simulink model "Application_BMS"  (R2024b)
settings: Solver=FixedStepDiscrete  StartTime=0.0  StopTime=660  FixedStep=BMSk_stepSize  RelTol=1e-3  EnableMultiTasking=on
values from neighbouring files (symbols this model uses):
  BMSc_airTemperature = air_temperature    (= 35)    [BMS_init.m]
  BMSc_cabinTemperature = 25    [BMS_init.m]
  BMSk_stepSize = 0.1    [BMS_init.m]
settings Model: PauseTimes=22  Creator=ms2zwt  LastModifiedBy=voillat
settings ConfigSet: Description=OpenECU configuration set for code generation under RTW-EC.
settings SolverCC: AlgebraicLoopSolver=TrustRegion  PositivePriorityOrder=on
settings DataIOCC: LimitDataPoints=on  SaveFormat=Array  SignalLoggingSaveFormat=ModelDataLogs
settings OptimizationCC: DefaultParameterBehavior=Inlined  InlineInvariantSignals=on  ExpressionDepthLimit=2147483647  StateBitsets=on  DataBitsets=on  ZeroExternalMemoryAtStartup=off  ZeroInternalMemoryAtStartup=off  NoFixptDivByZeroProtection=on  EfficientFloat2IntCast=on  LifeSpan=1  EfficientTunableParamExpr=on
settings DebuggingCC: SaveWithParameterizedLinksMsg=none  SignalResolutionControl=TryResolveAllWithWarning  MultiTaskDSMMsg=warning  MultiTaskCondExecSysMsg=none  SingleTaskRateTransMsg=error  CheckMatrixSingularityMsg=warning  VectorMatrixConversionMsg=warning  SignalLabelMismatchMsg=warning  UnconnectedInputMsg=warning  UnconnectedOutputMsg=warning  UnconnectedLineMsg=warning  AllowSymbolicDim=off  StateNameClashWarn=warning  SFUnexpectedBacktrackingDiag=warning  SFNoUnconditionalDefaultTransitionDiag=warning  SFExecutionAtInitializationDiag=none  ArithmeticOperatorsInVariantConditions=warning
settings HardwareCC: ProdBitPerPointer=32  ProdBitPerSizeT=32  ProdBitPerPtrDiffT=32  ProdLargestAtomicInteger=Long  ProdLargestAtomicFloat=Double  ProdEndianess=BigEndian  ProdWordSize=32  ProdHWDeviceType=Freescale->32-bit PowerPC  TargetIntDivRoundTo=Zero  TargetEndianess=BigEndian  TargetHWDeviceType=Freescale->32-bit PowerPC  ProdEqTarget=off
settings ModelReferenceCC: EnableRefExpFcnMdlSchedulingChecks=on  PropagateSignalLabelsOutOfModel=off
settings SFSimCC: SimUseLocalCustomCode=off  MATLABDynamicMemAlloc=off  CustomCodeUndefinedFunction=UseInterfaceOnly
settings RTWCC: Description=OpenECU Platform Target (ERT, optimised floating-point code)  SystemTargetFile=openecu_ert.tlc  MakeCommand=make_rtw optimized_floating_point=1  TemplateMakefile=openecu_ert_r2015b_64.tmf  RetainRTWFile=on  RTWUseLocalCustomCode=off  IncludeHyperlinkInReport=on  GPUComputeCapability=3.5
settings CodeAppCC: ForceParamTrailComments=on  IgnoreCustomStorageClasses=off  SimulinkDataObjDesc=on  CustomSymbolStrType=$N$R$M  InsertBlockDesc=on  StateflowObjectComments=on  InternalIdentifier=Classic
settings STFCustomTargetCC: TargetLibSuffix=.a  GenerateSampleERTMain=on  IncludeMdlTerminateFcn=off  CombineOutputUpdateFcns=on  IncludeFileDelimiter=UseQuote  ERTCustomFileBanners=on  SupportContinuousTime=off  RemoveResetFunc=on  MATLABClassNameForMDSCustomization=Simulink.SoftwareTarget.ERTCustomization  SystemTargetFile=openecu_ert.tlc
settings ERTTargetCC: MultiwordLength=2048  GenerateSampleERTMain=on  ParMdlRefBuildCompliant=off  CompOptLevelCompliant=off  ConcurrentExecutionCompliant=off  IncludeMdlTerminateFcn=off  IncludeFileDelimiter=UseQuote  SupportNonInlinedSFcns=on  ModelStepFunctionPrototypeControlCompliant=off  CPPClassGenCompliant=off  UseToolchainInfoCompliant=off  ExtModeMexFile=noextcomm  ERTSrcFileBannerTemplate=oe_code_c_template.cgt  ERTHdrFileBannerTemplate=oe_code_h_template.cgt  ERTDataSrcFileTemplate=oe_data_c_template.cgt  ERTDataHdrFileTemplate=oe_data_h_template.cgt  ERTCustomFileTemplate=example_file_process.tlc  GlobalDataDefinition=InSeparateSourceFile  GlobalDataReference=InSeparateHeaderFile  ConvertIfToSwitch=off  SuppressUnreachableDefaultCases=off  EnableUserReplacementTypes=on  DynamicArrayContainerType=coder::array
settings ConfigComp: CovMetricSettings=dw  CovSaveCumulativeToWorkspaceVar=on  CovSaveSingleToWorkspaceVar=on  CovExternalEMLEnable=off

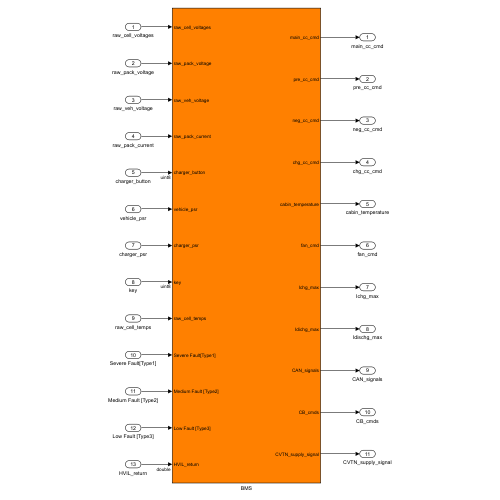
[thumbnail: Simulink's stored preview of the top-level diagram]
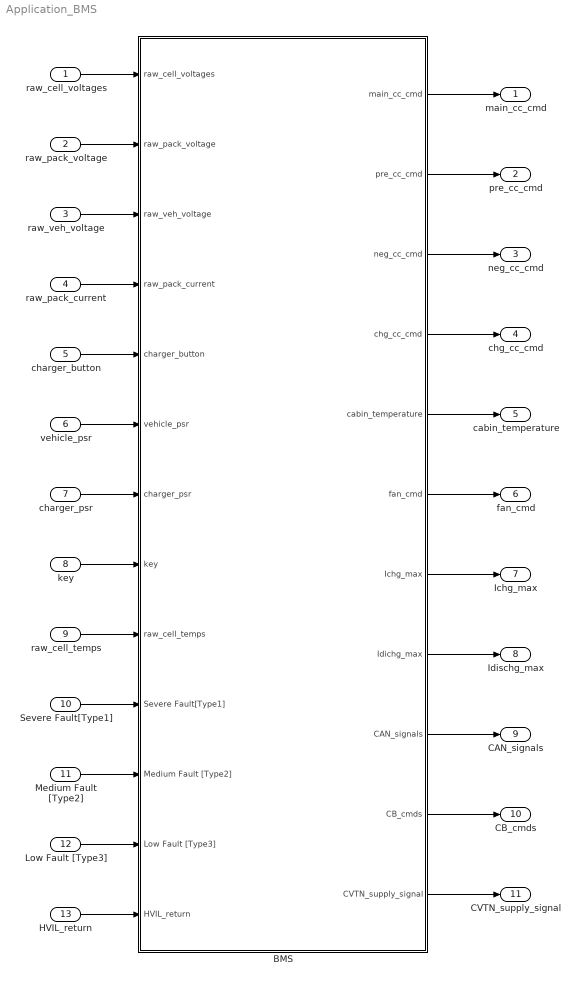
== system Application_BMS ==
  raw_cell_voltages : Inport
  raw_pack_voltage : Inport  Port=2
  raw_veh_voltage : Inport  Port=3
  raw_pack_current : Inport  Port=4
  charger_button : Inport  Port=5
  vehicle_psr : Inport  Port=6
  charger_psr : Inport  Port=7
  key : Inport  Port=8
  raw_cell_temps : Inport  Port=9
  Severe Fault[Type1] : Inport  Port=10
  Medium Fault [Type2] : Inport  Port=11
  Low Fault [Type3] : Inport  Port=12
  HVIL_return : Inport  Port=13
  BMS : Subsystem
  main_cc_cmd : Outport  VectorParamsAs1DForOutWhenUnconnected=off
  pre_cc_cmd : Outport  Port=2  VectorParamsAs1DForOutWhenUnconnected=off
  neg_cc_cmd : Outport  Port=3  VectorParamsAs1DForOutWhenUnconnected=off
  chg_cc_cmd : Outport  Port=4  VectorParamsAs1DForOutWhenUnconnected=off
  cabin_temperature : Outport  Port=5  VectorParamsAs1DForOutWhenUnconnected=off
  fan_cmd : Outport  Port=6  VectorParamsAs1DForOutWhenUnconnected=off
  Ichg_max : Outport  Port=7  VectorParamsAs1DForOutWhenUnconnected=off
  Idischg_max : Outport  Port=8  VectorParamsAs1DForOutWhenUnconnected=off
  CAN_signals : Outport  Port=9  VectorParamsAs1DForOutWhenUnconnected=off
  CB_cmds : Outport  Port=10  VectorParamsAs1DForOutWhenUnconnected=off
  CVTN_supply_signal : Outport  Port=11  VectorParamsAs1DForOutWhenUnconnected=off
  wires:
  raw_cell_voltages/1 -> BMS/1(raw_cell_voltages)
  raw_pack_voltage/1 -> BMS/2(raw_pack_voltage)
  raw_veh_voltage/1 -> BMS/3(raw_veh_voltage)
  raw_pack_current/1 -> BMS/4(raw_pack_current)
  charger_button/1 -> BMS/5(charger_button)
  vehicle_psr/1 -> BMS/6(vehicle_psr)
  charger_psr/1 -> BMS/7(charger_psr)
  key/1 -> BMS/8(key)
  raw_cell_temps/1 -> BMS/9(raw_cell_temps)
  Severe Fault[Type1]/1 -> BMS/10(Severe Fault[Type1])
  Medium Fault [Type2]/1 -> BMS/11(Medium Fault [Type2])
  Low Fault [Type3]/1 -> BMS/12(Low Fault [Type3])
  HVIL_return/1 -> BMS/13(HVIL_return)
  BMS/1(main_cc_cmd) -> main_cc_cmd/1
  BMS/2(pre_cc_cmd) -> pre_cc_cmd/1
  BMS/3(neg_cc_cmd) -> neg_cc_cmd/1
  BMS/4(chg_cc_cmd) -> chg_cc_cmd/1
  BMS/5(cabin_temperature) -> cabin_temperature/1
  BMS/6(fan_cmd) -> fan_cmd/1
  BMS/7(Ichg_max) -> Ichg_max/1
  BMS/8(Idichg_max) -> Idischg_max/1
  BMS/9(CAN_signals) -> CAN_signals/1
  BMS/10(CB_cmds) -> CB_cmds/1
  BMS/11(CVTN_supply_signal) -> CVTN_supply_signal/1

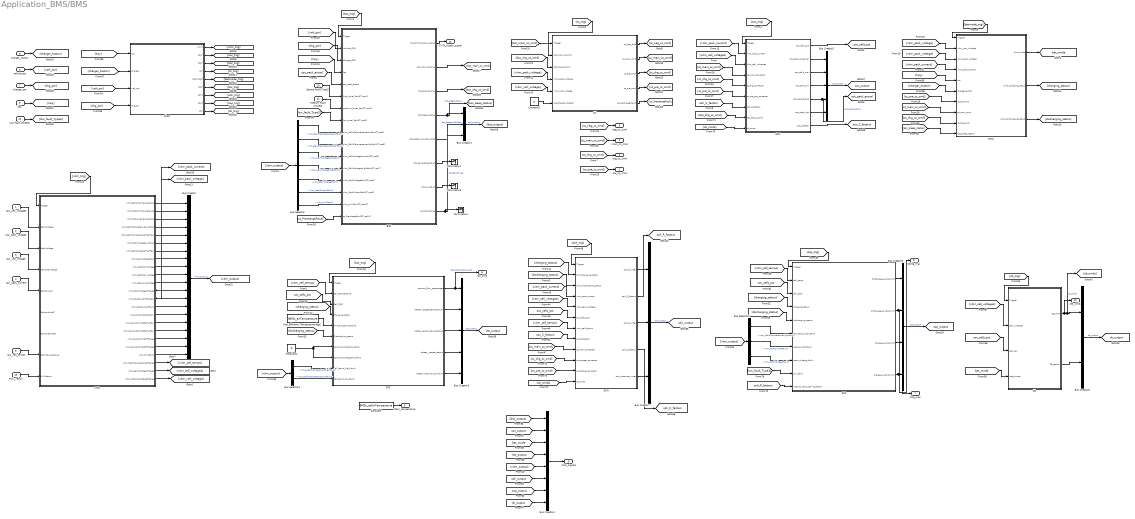
== system Application_BMS/BMS ==
  raw_cell_voltages : Inport
  raw_pack_voltage : Inport  Port=2
  raw_veh_voltage : Inport  Port=3
  raw_pack_current : Inport  Port=4
  charger_button : Inport  Port=5  OutDataTypeStr=uint8
  vehicle_psr : Inport  Port=6
  charger_psr : Inport  Port=7
  key : Inport  Port=8  OutDataTypeStr=uint8
  raw_cell_temps : Inport  Port=9
  Severe Fault[Type1] : Inport  Port=10
  Medium Fault [Type2] : Inport  Port=11
  Low Fault [Type3] : Inport  Port=12
  HVIL_return : Inport  Port=13  OutDataTypeStr=double
  BMO : Subsystem  Variant=on
  BSC : Subsystem  Variant=on
  BTC : Subsystem  Variant=on
  Bus Creator : BusCreator  Inputs=20
  Bus Creator1 : BusCreator  Inputs=3
  Bus Creator2 : BusCreator  Inputs=5
  Bus Creator3 : BusCreator  Inputs=5
  Bus Creator4 : BusCreator  Inputs=8
  Bus Creator5 : BusCreator  Inputs=4
  Bus Creator6 : BusCreator  Inputs=2
  Bus Creator7 : BusCreator  Inputs=3
  Bus Selector : BusSelector  OutputSignals=vitm_CellsTemperatureLowFault,vitm_CellsTemperatureHighFault,vitm_CellsVoltageLowFault,vitm_CellsVoltageHighFault,vitm_PackVoltageFault,vitm_PackCurrentFault,vitm_HVILFault
  Bus Selector1 : BusSelector  OutputSignals=vitm_CellsTemperatureHighFault,vitm_CellsTemperatureLowFault
  Bus Selector2 : BusSelector  OutputSignals=vitm_CellsTemperatureHighFault,vitm_PackCurrentFault,vitm_PackVoltageFault
  CB : Subsystem  Variant=on
  CC : Subsystem  Variant=on
  Chart : Stateflow chart  TreatAsAtomicUnit=on
  Constant : Constant  Value=BMSc_cabinTemperature  SampleTime=BMSk_stepSize
  Constant1 : Constant  Value=0  OutDataTypeStr=boolean  SampleTime=-1
  Constant2 : Constant  Value=0  OutDataTypeStr=double  SampleTime=-1
  Max Efficiency Temperature degC : Constant  Value=BMSc_airTemperature  SampleTime=BMSk_stepSize
  SOC : Subsystem  Variant=on
  SOH : Subsystem  Variant=on
  SOP : Subsystem  Variant=on
  Terminator1 : Terminator
  Terminator3 : Terminator
  Terminator4 : Terminator
  VITM : Subsystem  Variant=on
  main_cc_cmd : Outport  VectorParamsAs1DForOutWhenUnconnected=off
  pre_cc_cmd : Outport  Port=2  VectorParamsAs1DForOutWhenUnconnected=off
  neg_cc_cmd : Outport  Port=3  VectorParamsAs1DForOutWhenUnconnected=off
  chg_cc_cmd : Outport  Port=4  VectorParamsAs1DForOutWhenUnconnected=off
  cabin_temperature : Outport  Port=5  VectorParamsAs1DForOutWhenUnconnected=off
  fan_cmd : Outport  Port=6  VectorParamsAs1DForOutWhenUnconnected=off
  Ichg_max : Outport  Port=7  VectorParamsAs1DForOutWhenUnconnected=off
  Idichg_max : Outport  Port=8  VectorParamsAs1DForOutWhenUnconnected=off
  CAN_signals : Outport  Port=9  VectorParamsAs1DForOutWhenUnconnected=off
  CB_cmds : Outport  Port=10  VectorParamsAs1DForOutWhenUnconnected=off
  CVTN_supply_signal : Outport  Port=11  VectorParamsAs1DForOutWhenUnconnected=off
  tag scope: bat_mode=global, btc_output=global, cb_output=global, soc_C_factors=global, soc_cells_pct=global, soc_output=global, soc_pack_actual=global, soh_C_factors=global, soh_R_factors=global, soh_output=global, sop_output=global
  wires:
  Chart/1(vitm()) -> [vitm_trig]
  Chart/2(soc()) -> [soc_trig]
  Chart/3(bsc()) -> [bsc_trig]
  Chart/4(cc()) -> [cc_trig]
  Chart/5(batmode()) -> [batmode_trig]
  Constant/1 -> cabin_temperature/1
  [cc_neg_cc_cmd] -> neg_cc_cmd/1
  [cc_main_cc_cmd] -> main_cc_cmd/1
  [cc_chg_cc_cmd] -> chg_cc_cmd/1
  [cc_pre_cc_cmd] -> pre_cc_cmd/1
  Chart/6(btc()) -> [btc_trig]
  Bus Creator/1 -> [vitm_output]  "vitm_output"
  [vitm_output] -> Bus Selector/1
  charger_button/1 -> [charger_button]
  vehicle_psr/1 -> [veh_psr]
  [veh_psr] -> Chart/3(veh_psr)
  [vitm_output] -> Bus Selector1/1
  Bus Creator1/1 -> [bsc_output]  "bsc_output"
  Bus Creator2/1 -> [soc_output]  "soc_output"
  Bus Creator3/1 -> [btc_output]  "btc_output"
  [bsc_output] -> Bus Creator4/1
  [soc_output] -> Bus Creator4/2
  [bat_mode] -> Bus Creator4/3
  [btc_output] -> Bus Creator4/4
  [vitm_output] -> Bus Creator4/5
  Bus Creator4/1 -> CAN_signals/1
  Chart/7(soh()) -> [soh_trig]
  Chart/8(sop()) -> [sop_trig]
  [vitm_output] -> Bus Selector2/1
  Chart/9(cb()) -> [cb_trig]
  Bus Creator5/1 -> [sop_output]  "sop_output"
  [sop_output] -> Bus Creator4/7
  charger_psr/1 -> [chg_psr]
  [chg_psr] -> Chart/4(chg_psr)
  key/1 -> [key]
  [charger_button] -> Chart/2(charger)
  [key] -> Chart/1(key)
  Bus Creator6/1 -> [cb_output]  "cb_output"
  [cb_output] -> Bus Creator4/8
  Bus Creator7/1 -> [soh_output]  "soh_output"
  [soh_output] -> Bus Creator4/6
  Low Fault [Type3]/1 -> [low_fault_Type3]
  [vitm_pack_voltage] -> BMO/2(vitm_veh_voltage)
  [vitm_pack_voltage] -> BMO/3(vitm_pack_voltage)
  [vitm_pack_current] -> BMO/4(vitm_pack_current)
  [key] -> BMO/5(key)
  [charger_button] -> BMO/6(charger_button)
  [cc_pre_cc_cmd] -> BMO/7(cc_pre_cmd)
  [cc_main_cc_cmd] -> BMO/8(cc_main_cmd)
  [cc_chg_cc_cmd] -> BMO/9(cc_chg_cmd)
  [bsc_sleep_status] -> BMO/10(bsc_sleep_status)
  [batmode_trig] -> BMO/1(Trigger)
  BMO/1(bmo_mode) -> [bat_mode]
  BMO/2(bmo_charging_status) -> [charging_status]
  BMO/3(bmo_discharging_status) -> [discharging_status]
  [veh_psr] -> BSC/2(vehicle_PSR)
  [chg_psr] -> BSC/3(charger_PSR)
  [key] -> BSC/4(key)
  [soc_pack_actual] -> BSC/5(soc_pack_actual)
  Severe Fault[Type1]/1 -> BSC/6(high_level_fault[Type1])
  Medium Fault [Type2]/1 -> BSC/7(medium_level_fault[Type2])
  [low_fault_Type3] -> BSC/8(low_level_fault[Type3])
  Bus Selector/1 -> BSC/9(vitm_CellsTemperatureLowFault[Type4])  "<vitm_CellsTemperatureLowFault>"
  Bus Selector/2 -> BSC/10(vitm_CellsTemperatureHighFault[Type5])  "<vitm_CellsTemperatureHighFault>"
  Bus Selector/3 -> BSC/11(vitm_CellsVoltageLowFault[Type6])  "<vitm_CellsVoltageLowFault>"
  Bus Selector/4 -> BSC/12(vitm_CellsVoltageHightFault[Type7])  "<vitm_CellsVoltageHighFault>"
  Bus Selector/5 -> BSC/13(vitm_PackVoltageFault[Type8])  "<vitm_PackVoltageFault>"
  Bus Selector/6 -> BSC/14(vitm_PackCurrentFault[Type9])  "<vitm_PackCurrentFault>"
  Bus Selector/7 -> BSC/15(vitm_HVILFault[Type10])  "<vitm_HVILFault>"
  [cc_PrechargeFault] -> BSC/16(cc_PrechargeFault[Type11])
  [bsc_trig] -> BSC/1(Trigger)
  BSC/1(bsc_CVTN_supply_signal) -> CVTN_supply_signal/1
  BSC/2(bsc_main_cc_cmd) -> [bsc_main_cc_cmd]
  BSC/3(bsc_chg_cc_cmd) -> [bsc_chg_cc_cmd]
  BSC/4(bsc_sleep_status) -> Bus Creator1/1, [bsc_sleep_status]  "bsc_sleep_status"
  BSC/5(bsc_reason_to_open_CAN) -> Bus Creator1/2  "bsc_ReasonToOpen"
  BSC/6(bsc_severemed_fault) -> Terminator1/1
  BSC/7(bsc_low_fault) -> Terminator3/1
  BSC/8(bsc_fault_type) -> Terminator4/1, Bus Creator1/3  "bsc_FaultType"
  [vitm_cell_temps] -> BTC/2(Cell_temperature)
  [soc_cells_pct] -> BTC/3(Cell_SOC)
  [charging_status] -> BTC/4(Charging_status)
  Max Efficiency Temperature degC/1 -> BTC/5(Ambient_temperature)
  [discharging_status] -> BTC/6(Discharging_status)
  Constant1/1 -> BTC/7(Coolant_inlet_temp_fault), BTC/8(Coolant_outlet_temp_fault)
  Bus Selector1/1 -> BTC/9(Cell_temp_high_fault)  "<vitm_CellsTemperatureHighFault>"
  Bus Selector1/2 -> BTC/10(Cell_temp_low_fault)  "<vitm_CellsTemperatureLowFault>"
  [btc_trig] -> BTC/1(Trigger)
  BTC/1(coolant_flow_percentage) -> Bus Creator3/1, fan_cmd/1  "btc_coolant_flow_pct"
  BTC/2(battery_target_temperature) -> Bus Creator3/2
  BTC/3(battery_actual_temperature) -> Bus Creator3/3
  BTC/4(battery_reqest_status) -> Bus Creator3/4
  BTC/5(battery_thermal_condition) -> Bus Creator3/5
  [vitm_cell_voltages] -> CB/2(cell_voltages)
  [soc_cells_pct] -> CB/3(cell_soc)
  [bat_mode] -> CB/4(batt_mode)
  [cb_trig] -> CB/1(Trigger)
  CB/1(CB_cmd) -> [cb_cmds], Bus Creator6/1, CB_cmds/1  "cb_cmds"
  CB/2(CB_status) -> Bus Creator6/2
  [bsc_main_cc_cmd] -> CC/2(bsc_main_cc_cmd)
  [bsc_chg_cc_cmd] -> CC/3(bsc_chg_cc_cmd)
  [vitm_pack_voltage] -> CC/4(vitm_pack_voltage)
  [vitm_veh_voltage] -> CC/5(vitm_veh_voltage)
  Constant2/1 -> CC/6(pre_chg_fault_reset)
  [cc_trig] -> CC/1(Trigger)
  CC/1(cc_neg_cmd) -> [cc_neg_cc_cmd]
  CC/2(cc_main_cmd) -> [cc_main_cc_cmd]
  CC/3(cc_chg_cmd) -> [cc_chg_cc_cmd]
  CC/4(cc_pre_cmd) -> [cc_pre_cc_cmd]
  CC/5(cc_precharge_fault) -> [cc_PrechargeFault]
  [vitm_pack_current] -> SOC/2(vitm_pack_current)
  [vitm_cell_voltages] -> SOC/3(vitm_cell_voltages)
  [cc_main_cc_cmd] -> SOC/4(cc_main_contactor)
  [cc_chg_cc_cmd] -> SOC/5(cc_chg_contactor)
  [cc_pre_cc_cmd] -> SOC/6(cc_pre_chg_contactor)
  [soh_C_factors] -> SOC/7(soh_C_factors)
  [bsc_chg_cc_cmd] -> SOC/8(bsc_chg_cc_cmd)
  [cb_cmds] -> SOC/9(cb_cmds)
  [soc_trig] -> SOC/1(Trigger)
  SOC/1(soc_cells_pct) -> [soc_cells_pct]
  SOC/2(soc_pack_customer) -> Bus Creator2/1
  SOC/3(soc_cells_max) -> Bus Creator2/2
  SOC/4(soc_cells_min) -> Bus Creator2/3
  SOC/5(soc_pack_actual) -> [soc_pack_actual], Bus Creator2/4  "soc_pack_actual"
  SOC/6(soc_rate_high) -> Bus Creator2/5
  SOC/7(soc_C_factor) -> [soc_C_factors]
  [charging_status] -> SOH/2(bmo_charging_status)
  [discharging_status] -> SOH/3(bmo_discharging_status)
  [vitm_pack_current] -> SOH/4(vitm_pack_current)
  [vitm_cell_voltages] -> SOH/5(vitm_cell_voltages)
  [soc_cells_pct] -> SOH/6(soc_cells_pct)
  [vitm_cell_temps] -> SOH/7(vitm_cells_temp)
  [soc_C_factors] -> SOH/8(soc_C_factors)
  [cc_main_cc_cmd] -> SOH/9(cc_main_contactor)
  [cc_chg_cc_cmd] -> SOH/10(cc_charger_contactor)
  [cc_pre_cc_cmd] -> SOH/11(cc_prechg_contactor)
  [cb_cmds] -> SOH/12(cb_cmds)
  [soh_trig] -> SOH/1(Trigger)
  SOH/1(soh_R_index) -> Bus Creator7/1
  SOH/2(soh_R_factors) -> [soh_R_factors]
  SOH/3(soh_C_index) -> Bus Creator7/2
  SOH/4(soh_C_factors) -> [soh_C_factors]
  SOH/5(soh_customer_index) -> Bus Creator7/3
  [vitm_cell_temps] -> SOP/2(cell_temp)
  [soc_cells_pct] -> SOP/3(cell_SOC)
  [charging_status] -> SOP/4(charging_status)
  [discharging_status] -> SOP/5(discharging_status)
  Bus Selector2/1 -> SOP/6(cell_temp_high_Fault)  "<vitm_CellsTemperatureHighFault>"
  Bus Selector2/2 -> SOP/7(pack_current_fault)  "<vitm_PackCurrentFault>"
  Bus Selector2/3 -> SOP/8(pack_voltage_fault)  "<vitm_PackVoltageFault>"
  [low_fault_Type3] -> SOP/9(low_fault)
  [soh_R_factors] -> SOP/10(internal_resis_scaling_factor)
  [sop_trig] -> SOP/1(Trigger)
  SOP/1(discharge_power_limit) -> Bus Creator5/1
  SOP/2(discharge_current_limit) -> Idichg_max/1, Bus Creator5/2
  SOP/3(charge_power_limit) -> Bus Creator5/3
  SOP/4(charge_current_limit) -> Bus Creator5/4, Ichg_max/1
  raw_cell_voltages/1 -> VITM/2(CellVoltages)
  raw_pack_voltage/1 -> VITM/3(PackVoltage)
  raw_veh_voltage/1 -> VITM/4(VehSideVoltage)
  raw_pack_current/1 -> VITM/5(PackCurrent)
  raw_cell_temps/1 -> VITM/8(CellsTemperature)
  HVIL_return/1 -> VITM/9(HVILReturn)
  [vitm_trig] -> VITM/1(Trigger)
  VITM/1(vitm_CellsMaxTemperature) -> Bus Creator/1
  VITM/2(vitm_CellsMinTemperature) -> Bus Creator/2
  VITM/3(vitm_CellsAvgTemperature) -> Bus Creator/3
  VITM/4(vitm_CellsTemperatureLowFault) -> Bus Creator/4
  VITM/5(vitm_CellsTemperatureHighFault) -> Bus Creator/5
  VITM/6(vitm_CellsVoltageLowFault) -> Bus Creator/6
  VITM/7(vitm_CellsVoltageHighFault) -> Bus Creator/7
  VITM/8(vitm_PackVoltageFault) -> Bus Creator/8
  VITM/9(vitm_CellsMinVoltage) -> Bus Creator/9
  VITM/10(vitm_CellsMaxVoltage) -> Bus Creator/10
  VITM/11(vitm_CellsAvgVoltage) -> Bus Creator/11
  VITM/12(vitm_PackVoltageFiltered) -> Bus Creator/12, [vitm_pack_voltage]
  VITM/13(vitm_PackCurrentFiltered) -> Bus Creator/13, [vitm_pack_current]
  VITM/14(vitm_PackCurrentFault) -> Bus Creator/14
  VITM/15(vitm_CoolantDeltaTemp) -> Bus Creator/15
  VITM/16(vitm_CoolantInletTempFault) -> Bus Creator/16
  VITM/17(vitm_CoolantOutlletTempFault) -> Bus Creator/17
  VITM/18(vitm_CoolantInletTFiltered) -> Bus Creator/18
  VITM/19(vitm_CoolantOutletTFiltered) -> Bus Creator/19
  VITM/20(vitm_HVILFault) -> Bus Creator/20
  VITM/21(vitm_CellsTemperatureFiltered) -> [vitm_cell_temps]
  VITM/22(vitm_CellsVoltageFiltered) -> [vitm_cell_voltages]
  VITM/23(vitm_VehSideVoltageFiltered) -> [vitm_veh_voltage]

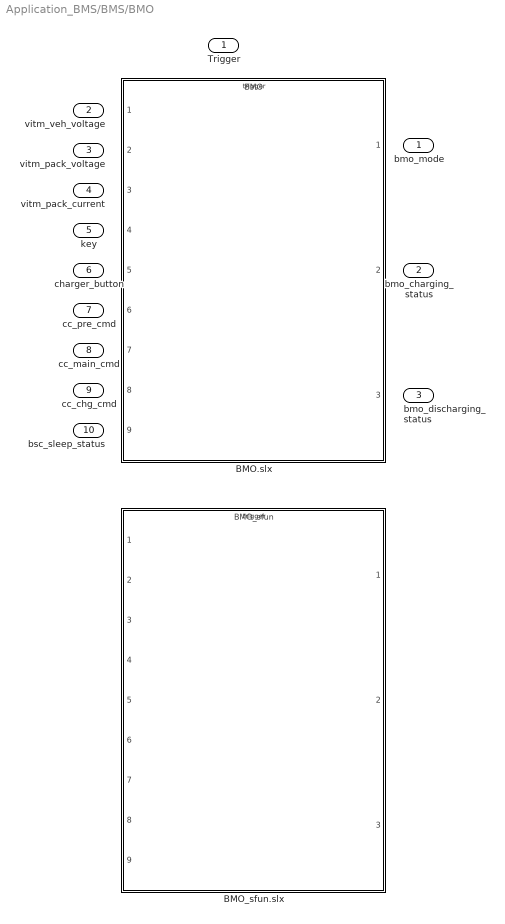
== system Application_BMS/BMS/BMO ==
  Trigger : Inport
  vitm_veh_voltage : Inport  Port=2
  vitm_pack_voltage : Inport  Port=3
  vitm_pack_current : Inport  Port=4
  key : Inport  Port=5
  charger_button : Inport  Port=6
  cc_pre_cmd : Inport  Port=7
  cc_main_cmd : Inport  Port=8
  cc_chg_cmd : Inport  Port=9
  bsc_sleep_status : Inport  Port=10
  BMO.slx : ModelReference  ModelNameDialog=BMO.slx  SimulationMode=Normal  VariantControl=use_bmo_sfun == 0  ModelReferenceVersion=15.2  TriggerPortName=Trigger  TriggerPortTriggerType=function-call  TriggerPortStatesWhenEnabling=held
  BMO_sfun.slx : ModelReference  ModelNameDialog=BMO_sfun.slx  SimulationMode=Normal  VariantControl=use_bmo_sfun == 1  ModelReferenceVersion=19.2  TriggerPortName=Trigger  TriggerPortTriggerType=function-call  TriggerPortStatesWhenEnabling=held
  bmo_mode : Outport
  bmo_charging_status : Outport  Port=2
  bmo_discharging_status : Outport  Port=3

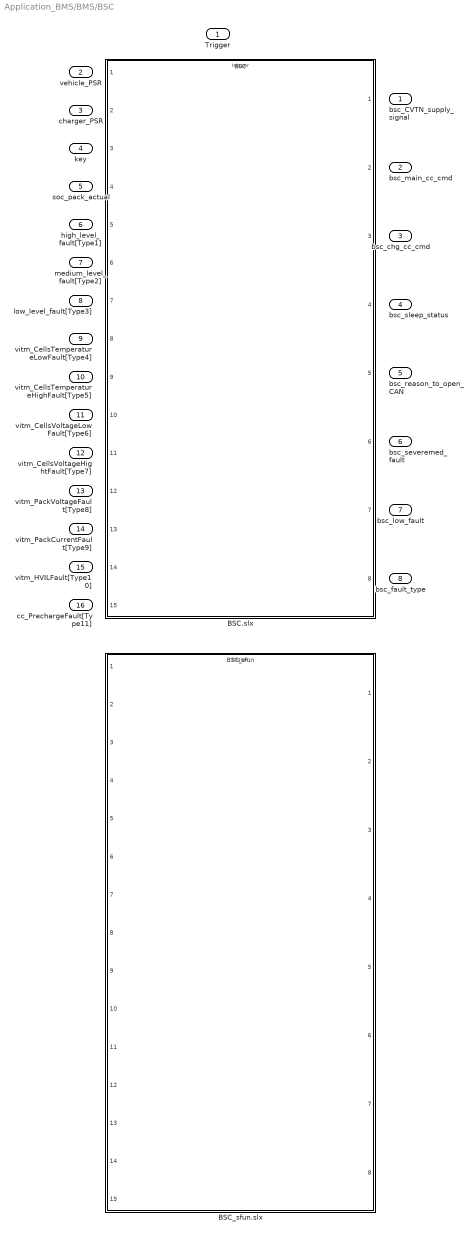
== system Application_BMS/BMS/BSC ==
  Trigger : Inport
  vehicle_PSR : Inport  Port=2
  charger_PSR : Inport  Port=3
  key : Inport  Port=4
  soc_pack_actual : Inport  Port=5
  high_level_fault[Type1] : Inport  Port=6
  medium_level_fault[Type2] : Inport  Port=7
  low_level_fault[Type3] : Inport  Port=8
  vitm_CellsTemperatureLowFault[Type4] : Inport  Port=9
  vitm_CellsTemperatureHighFault[Type5] : Inport  Port=10
  vitm_CellsVoltageLowFault[Type6] : Inport  Port=11
  vitm_CellsVoltageHightFault[Type7] : Inport  Port=12
  vitm_PackVoltageFault[Type8] : Inport  Port=13
  vitm_PackCurrentFault[Type9] : Inport  Port=14
  vitm_HVILFault[Type10] : Inport  Port=15
  cc_PrechargeFault[Type11] : Inport  Port=16
  BSC.slx : ModelReference  ModelNameDialog=BSC.slx  SimulationMode=Normal  VariantControl=use_bsc_sfun == 0  ModelReferenceVersion=15.2  TriggerPortName=Trigger  TriggerPortTriggerType=function-call  TriggerPortStatesWhenEnabling=held
  BSC_sfun.slx : ModelReference  ModelNameDialog=BSC_sfun.slx  SimulationMode=Normal  VariantControl=use_bsc_sfun == 1  ModelReferenceVersion=19.2  TriggerPortName=Trigger  TriggerPortTriggerType=function-call  TriggerPortStatesWhenEnabling=held
  bsc_CVTN_supply_signal : Outport
  bsc_main_cc_cmd : Outport  Port=2
  bsc_chg_cc_cmd : Outport  Port=3
  bsc_sleep_status : Outport  Port=4
  bsc_reason_to_open_CAN : Outport  Port=5
  bsc_severemed_fault : Outport  Port=6
  bsc_low_fault : Outport  Port=7
  bsc_fault_type : Outport  Port=8

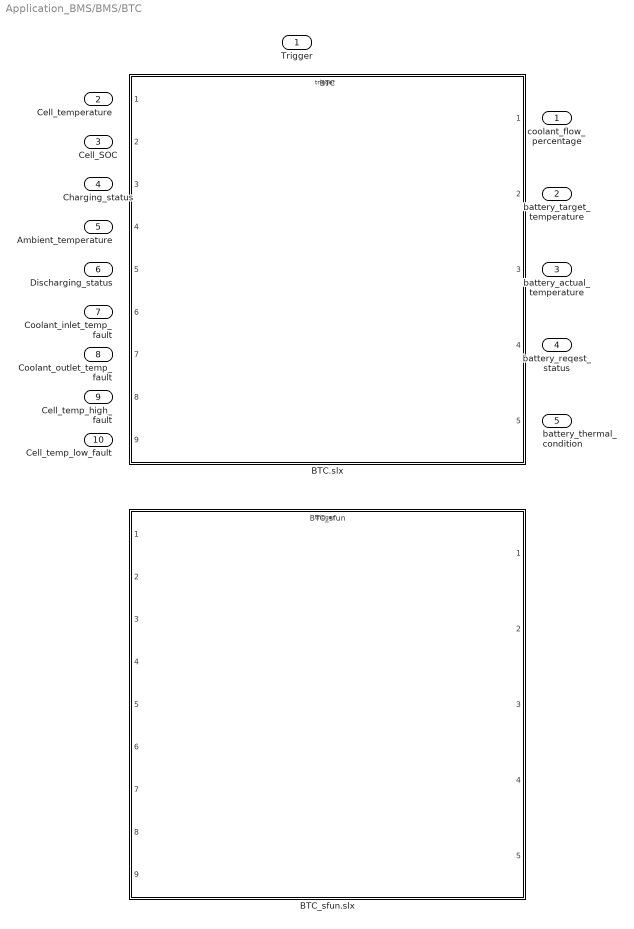
== system Application_BMS/BMS/BTC ==
  Trigger : Inport
  Cell_temperature : Inport  Port=2
  Cell_SOC : Inport  Port=3
  Charging_status : Inport  Port=4
  Ambient_temperature : Inport  Port=5
  Discharging_status : Inport  Port=6
  Coolant_inlet_temp_fault : Inport  Port=7
  Coolant_outlet_temp_fault : Inport  Port=8
  Cell_temp_high_fault : Inport  Port=9
  Cell_temp_low_fault : Inport  Port=10
  BTC.slx : ModelReference  ModelNameDialog=BTC.slx  SimulationMode=Normal  VariantControl=use_btc_sfun == 0  ModelReferenceVersion=15.2  TriggerPortName=Trigger  TriggerPortTriggerType=function-call  TriggerPortStatesWhenEnabling=held
  BTC_sfun.slx : ModelReference  ModelNameDialog=BTC_sfun.slx  SimulationMode=Normal  VariantControl=use_btc_sfun == 1  ModelReferenceVersion=19.2  TriggerPortName=Trigger  TriggerPortTriggerType=function-call  TriggerPortStatesWhenEnabling=held
  coolant_flow_percentage : Outport
  battery_target_temperature : Outport  Port=2
  battery_actual_temperature : Outport  Port=3
  battery_reqest_status : Outport  Port=4
  battery_thermal_condition : Outport  Port=5

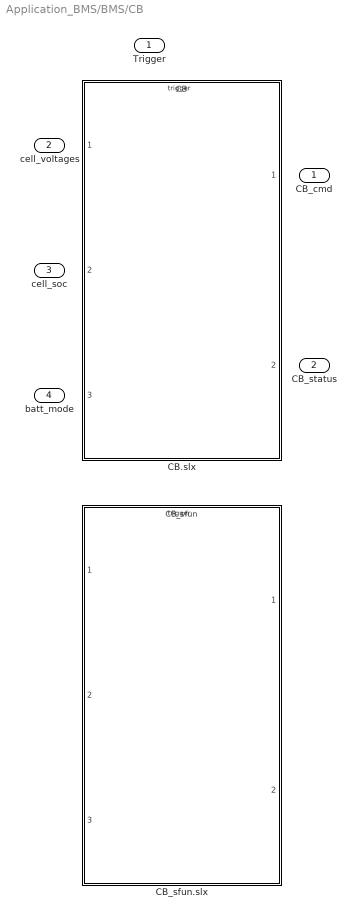
== system Application_BMS/BMS/CB ==
  Trigger : Inport
  cell_voltages : Inport  Port=2
  cell_soc : Inport  Port=3
  batt_mode : Inport  Port=4
  CB.slx : ModelReference  ModelNameDialog=CB.slx  SimulationMode=Normal  VariantControl=use_cb_sfun == 0  ModelReferenceVersion=15.1  TriggerPortName=Trigger  TriggerPortTriggerType=function-call  TriggerPortStatesWhenEnabling=held
  CB_sfun.slx : ModelReference  ModelNameDialog=CB_sfun.slx  SimulationMode=Normal  VariantControl=use_cb_sfun == 1  ModelReferenceVersion=19.2  TriggerPortName=Trigger  TriggerPortTriggerType=function-call  TriggerPortStatesWhenEnabling=held
  CB_cmd : Outport
  CB_status : Outport  Port=2

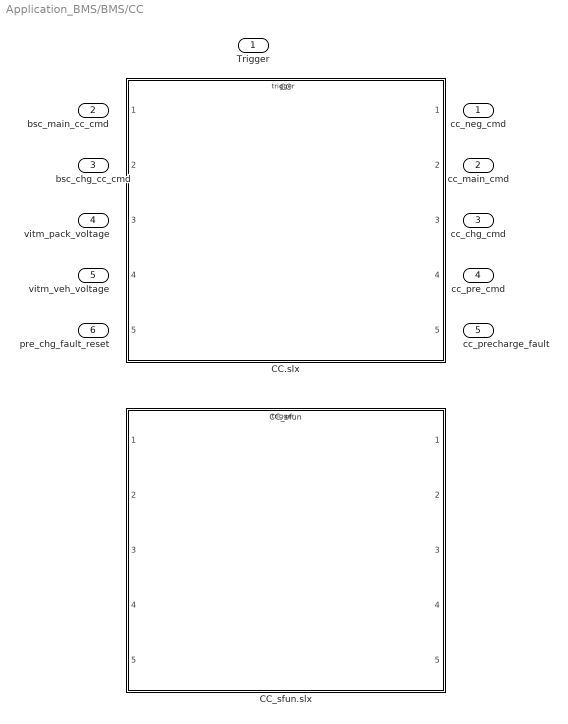
== system Application_BMS/BMS/CC ==
  Trigger : Inport
  bsc_main_cc_cmd : Inport  Port=2
  bsc_chg_cc_cmd : Inport  Port=3
  vitm_pack_voltage : Inport  Port=4
  vitm_veh_voltage : Inport  Port=5
  pre_chg_fault_reset : Inport  Port=6
  CC.slx : ModelReference  ModelNameDialog=CC.slx  SimulationMode=Normal  VariantControl=use_cc_sfun == 0  ModelReferenceVersion=15.2  TriggerPortName=Trigger  TriggerPortTriggerType=function-call  TriggerPortStatesWhenEnabling=held
  CC_sfun.slx : ModelReference  ModelNameDialog=CC_sfun.slx  SimulationMode=Normal  VariantControl=use_cc_sfun == 1  ModelReferenceVersion=19.2  TriggerPortName=Trigger  TriggerPortTriggerType=function-call  TriggerPortStatesWhenEnabling=held
  cc_neg_cmd : Outport
  cc_main_cmd : Outport  Port=2
  cc_chg_cmd : Outport  Port=3
  cc_pre_cmd : Outport  Port=4
  cc_precharge_fault : Outport  Port=5

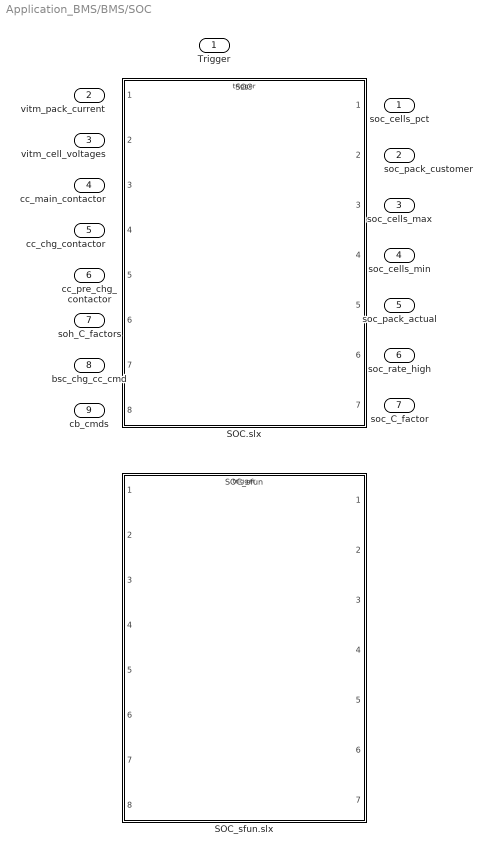
== system Application_BMS/BMS/SOC ==
  Trigger : Inport
  vitm_pack_current : Inport  Port=2
  vitm_cell_voltages : Inport  Port=3
  cc_main_contactor : Inport  Port=4
  cc_chg_contactor : Inport  Port=5
  cc_pre_chg_contactor : Inport  Port=6
  soh_C_factors : Inport  Port=7
  bsc_chg_cc_cmd : Inport  Port=8
  cb_cmds : Inport  Port=9
  SOC.slx : ModelReference  ModelNameDialog=SOC.slx  SimulationMode=Normal  VariantControl=use_soc_sfun == 0  ModelReferenceVersion=15.2  TriggerPortName=Trigger  TriggerPortTriggerType=function-call  TriggerPortStatesWhenEnabling=held
  SOC_sfun.slx : ModelReference  ModelNameDialog=SOC_sfun.slx  SimulationMode=Normal  VariantControl=use_soc_sfun == 1  ModelReferenceVersion=19.2  TriggerPortName=Trigger  TriggerPortTriggerType=function-call  TriggerPortStatesWhenEnabling=held
  soc_cells_pct : Outport
  soc_pack_customer : Outport  Port=2
  soc_cells_max : Outport  Port=3
  soc_cells_min : Outport  Port=4
  soc_pack_actual : Outport  Port=5
  soc_rate_high : Outport  Port=6
  soc_C_factor : Outport  Port=7

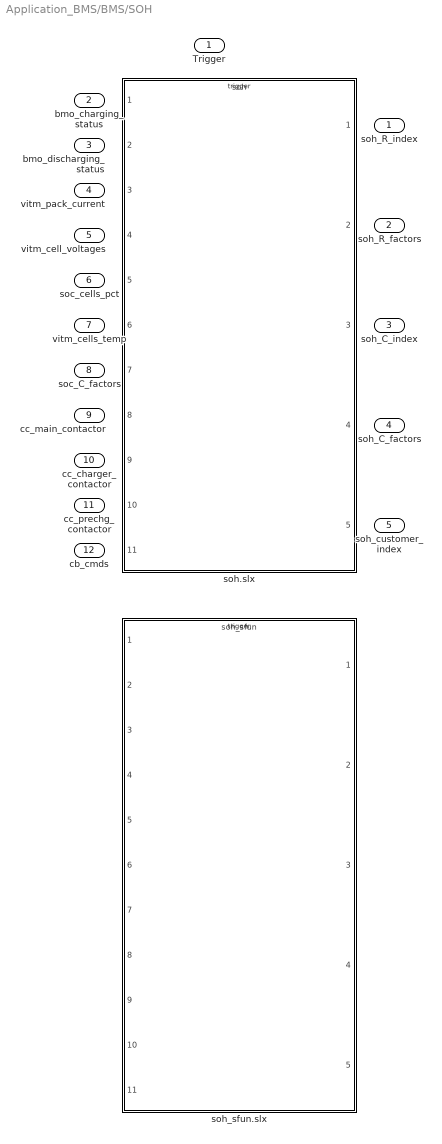
== system Application_BMS/BMS/SOH ==
  Trigger : Inport
  bmo_charging_status : Inport  Port=2
  bmo_discharging_status : Inport  Port=3
  vitm_pack_current : Inport  Port=4
  vitm_cell_voltages : Inport  Port=5
  soc_cells_pct : Inport  Port=6
  vitm_cells_temp : Inport  Port=7
  soc_C_factors : Inport  Port=8
  cc_main_contactor : Inport  Port=9
  cc_charger_contactor : Inport  Port=10
  cc_prechg_contactor : Inport  Port=11
  cb_cmds : Inport  Port=12
  soh.slx : ModelReference  ModelNameDialog=soh.slx  SimulationMode=Normal  VariantControl=use_soh_sfun == 0  ModelReferenceVersion=15.2  TriggerPortName=Trigger  TriggerPortTriggerType=function-call  TriggerPortStatesWhenEnabling=held
  soh_sfun.slx : ModelReference  ModelNameDialog=soh_sfun.slx  SimulationMode=Normal  VariantControl=use_soh_sfun == 1  ModelReferenceVersion=19.2  TriggerPortName=Trigger  TriggerPortTriggerType=function-call  TriggerPortStatesWhenEnabling=held
  soh_R_index : Outport
  soh_R_factors : Outport  Port=2
  soh_C_index : Outport  Port=3
  soh_C_factors : Outport  Port=4
  soh_customer_index : Outport  Port=5

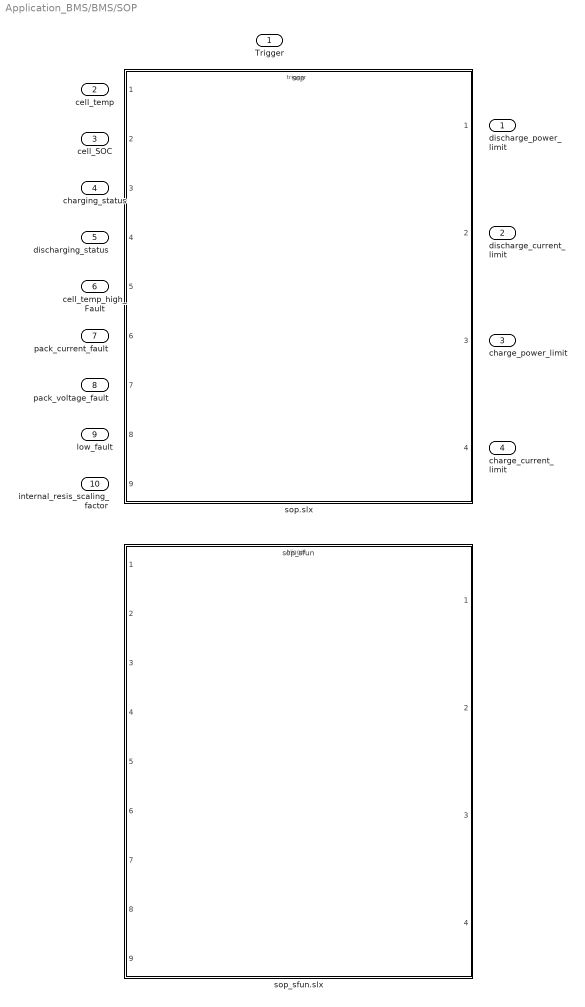
== system Application_BMS/BMS/SOP ==
  Trigger : Inport
  cell_temp : Inport  Port=2
  cell_SOC : Inport  Port=3
  charging_status : Inport  Port=4
  discharging_status : Inport  Port=5
  cell_temp_high_Fault : Inport  Port=6
  pack_current_fault : Inport  Port=7
  pack_voltage_fault : Inport  Port=8
  low_fault : Inport  Port=9
  internal_resis_scaling_factor : Inport  Port=10
  sop.slx : ModelReference  ModelNameDialog=sop.slx  SimulationMode=Normal  VariantControl=use_sop_sfun == 0  ModelReferenceVersion=15.2  TriggerPortName=Trigger  TriggerPortTriggerType=function-call  TriggerPortStatesWhenEnabling=held
  sop_sfun.slx : ModelReference  ModelNameDialog=sop_sfun.slx  SimulationMode=Normal  VariantControl=use_sop_sfun == 1  ModelReferenceVersion=19.2  TriggerPortName=Trigger  TriggerPortTriggerType=function-call  TriggerPortStatesWhenEnabling=held
  discharge_power_limit : Outport
  discharge_current_limit : Outport  Port=2
  charge_power_limit : Outport  Port=3
  charge_current_limit : Outport  Port=4

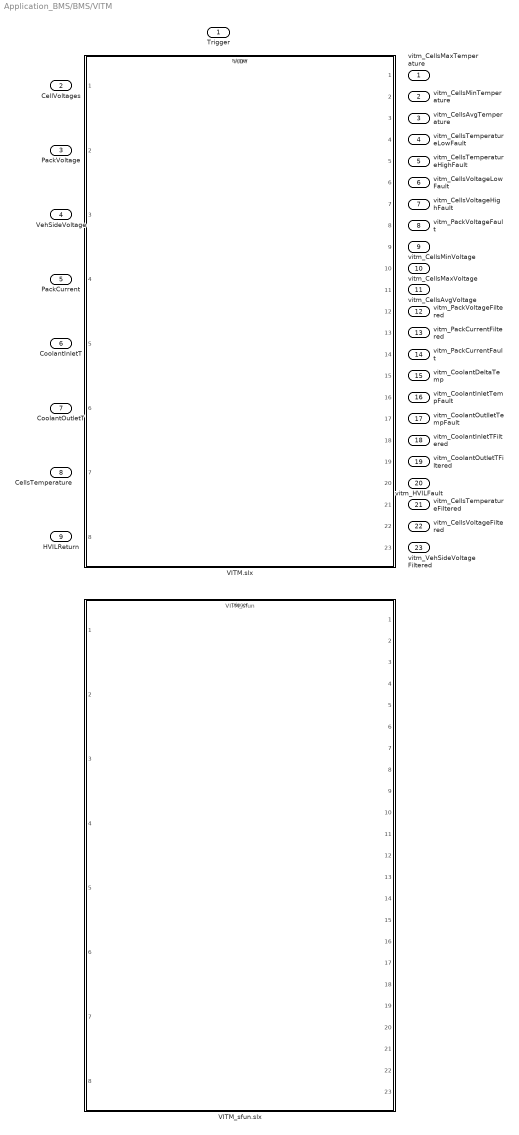
== system Application_BMS/BMS/VITM ==
  Trigger : Inport
  CellVoltages : Inport  Port=2
  PackVoltage : Inport  Port=3
  VehSideVoltage : Inport  Port=4
  PackCurrent : Inport  Port=5
  CoolantInletT : Inport  Port=6
  CoolantOutletT : Inport  Port=7
  CellsTemperature : Inport  Port=8
  HVILReturn : Inport  Port=9
  VITM.slx : ModelReference  ModelNameDialog=VITM.slx  SimulationMode=Normal  VariantControl=use_vit_sfun == 0  ModelReferenceVersion=15.1  TriggerPortName=Trigger  TriggerPortTriggerType=function-call  TriggerPortStatesWhenEnabling=held
  VITM_sfun.slx : ModelReference  ModelNameDialog=VITM_sfun.slx  SimulationMode=Normal  VariantControl=use_vit_sfun == 1  ModelReferenceVersion=19.2  TriggerPortName=Trigger  TriggerPortTriggerType=function-call  TriggerPortStatesWhenEnabling=held
  vitm_CellsMaxTemperature : Outport
  vitm_CellsMinTemperature : Outport  Port=2
  vitm_CellsAvgTemperature : Outport  Port=3
  vitm_CellsTemperatureLowFault : Outport  Port=4
  vitm_CellsTemperatureHighFault : Outport  Port=5
  vitm_CellsVoltageLowFault : Outport  Port=6
  vitm_CellsVoltageHighFault : Outport  Port=7
  vitm_PackVoltageFault : Outport  Port=8
  vitm_CellsMinVoltage : Outport  Port=9
  vitm_CellsMaxVoltage : Outport  Port=10
  vitm_CellsAvgVoltage : Outport  Port=11
  vitm_PackVoltageFiltered : Outport  Port=12
  vitm_PackCurrentFiltered : Outport  Port=13
  vitm_PackCurrentFault : Outport  Port=14
  vitm_CoolantDeltaTemp : Outport  Port=15
  vitm_CoolantInletTempFault : Outport  Port=16
  vitm_CoolantOutlletTempFault : Outport  Port=17
  vitm_CoolantInletTFiltered : Outport  Port=18
  vitm_CoolantOutletTFiltered : Outport  Port=19
  vitm_HVILFault : Outport  Port=20
  vitm_CellsTemperatureFiltered : Outport  Port=21
  vitm_CellsVoltageFiltered : Outport  Port=22
  vitm_VehSideVoltageFiltered : Outport  Port=23

== stateflow chart Application_BMS/BMS/Chart ==
  state main_chg
    (default) -> (junction 607)
    main_chg -> (junction 607) [order 1]
    (junction 607) -> (junction 606) : {vitm;}
    (junction 606) -> (junction 597) : {soc;}
    (junction 597) -> (junction 612) : {bsc;}
    (junction 612) -> (junction 598) : {soh;}
    (junction 598) -> (junction 604) : {cc;}
    (junction 604) -> (junction 605) : {batmode;}
    (junction 605) -> (junction 592) : {btc;}
    (junction 592) -> (junction 593) : {sop;}
    (junction 593) -> (junction 594) : {cb;}
  state main_key
    (default) -> (junction 544)
    main_key -> (junction 544) [order 1]
    (junction 544) -> (junction 543) : {vitm;}
    (junction 543) -> (junction 534) : {soc;}
    (junction 534) -> (junction 549) : {bsc;}
    (junction 549) -> (junction 535) : {soh;}
    (junction 535) -> (junction 541) : {cc;}
    (junction 541) -> (junction 542) : {batmode;}
    (junction 542) -> (junction 529) : {btc;}
    (junction 529) -> (junction 530) : {sop;}
    (junction 530) -> (junction 531) : {cb;}
  state init_key
    (default) -> (junction 81)
    init_key -> (junction 81) [order 1]
    (junction 81) -> (junction 83) : {vitm;}
    (junction 83) -> (junction 89) : {soc;}
    (junction 89) -> (junction 527) : {bsc;}
    (junction 527) -> (junction 82) : {soh;}
    (junction 82) -> (junction 85) : {cc;}
    (junction 85) -> (junction 87) : {batmode;}
    (junction 87) -> (junction 158) : {btc;}
    (junction 158) -> (junction 195) : {sop;}
    (junction 195) -> (junction 236) : {cb;}
  state init_chg
    (default) -> (junction 586)
    init_chg -> (junction 586) [order 1]
    (junction 586) -> (junction 585) : {vitm;}
    (junction 585) -> (junction 576) : {soc;}
    (junction 576) -> (junction 591) : {bsc;}
    (junction 591) -> (junction 577) : {soh;}
    (junction 577) -> (junction 583) : {cc;}
    (junction 583) -> (junction 584) : {batmode;}
    (junction 584) -> (junction 571) : {btc;}
    (junction 571) -> (junction 572) : {sop;}
    (junction 572) -> (junction 573) : {cb;}
  state no_power
    entry:
    end_count =0;
  state end_key
    exit:
    end_count = end_count +1;
    (default) -> (junction 565)
    end_key -> (junction 565) [order 1]
    (junction 565) -> (junction 564) : {vitm;}
    (junction 564) -> (junction 555) : {soc;}
    (junction 555) -> (junction 570) : {bsc;}
    (junction 570) -> (junction 556) : {soh;}
    (junction 556) -> (junction 562) : {cc;}
    (junction 562) -> (junction 563) : {batmode;}
    (junction 563) -> (junction 550) : {btc;}
    (junction 550) -> (junction 551) : {sop;}
    (junction 551) -> (junction 552) : {cb;}
  state end_chg
    exit:
    end_count = end_count +1;
    (default) -> (junction 628)
    end_chg -> (junction 628) [order 1]
    (junction 628) -> (junction 627) : {vitm;}
    (junction 627) -> (junction 618) : {soc;}
    (junction 618) -> (junction 633) : {bsc;}
    (junction 633) -> (junction 619) : {soh;}
    (junction 619) -> (junction 625) : {cc;}
    (junction 625) -> (junction 626) : {batmode;}
    (junction 626) -> (junction 613) : {btc;}
    (junction 613) -> (junction 614) : {sop;}
    (junction 614) -> (junction 615) : {cb;}
  (default) -> no_power
  no_power -> init_chg [order 2] : [charger > 0.5]
  no_power -> init_key [order 1] : [key > 0.5]
  end_chg -> no_power [order 2]
  end_key -> no_power [order 2]
  init_key -> main_key [order 1]
  init_chg -> main_chg [order 1]
  main_chg -> end_chg [order 1] : [chg_psr < 0.5]
  main_key -> end_key [order 1] : [veh_psr < 0.5]
  end_key -> end_key [order 1] : [end_count < 10]
  end_chg -> end_chg [order 1] : [end_count < 10]
  data: key input; charger input; veh_psr input; end_count local double =0; chg_psr input
  events: vitm output FUNCTION_CALL_EVENT; soc output FUNCTION_CALL_EVENT; bsc output FUNCTION_CALL_EVENT; cc output FUNCTION_CALL_EVENT; batmode output FUNCTION_CALL_EVENT; btc output FUNCTION_CALL_EVENT; soh output FUNCTION_CALL_EVENT; sop output FUNCTION_CALL_EVENT; cb output FUNCTION_CALL_EVENT
